simulink model "Polaris_demo"  (Simulink 9.2)
settings: Solver=FixedStepDiscrete  StartTime=0.0  StopTime=Inf  RelTol=1e-3  EnableMultiTasking=on
libraries: rpi_blkst x2
settings Model: Creator=jacques  LastModifiedBy=jacques  SimulationMode=external
settings OptimizationCC: ExpressionDepthLimit=2147483647  LifeSpan=1
settings DebuggingCC: SolverPrmCheckMsg=warning
settings HardwareCC: ProdLargestAtomicInteger=Long  ProdLargestAtomicFloat=Double  ProdIntDivRoundTo=Zero  ProdEndianess=LittleEndian  ProdHWDeviceType=ARM Compatible->ARM Cortex
settings SFSimCC: MATLABDynamicMemAlloc=off
settings RTWCC: SystemTargetFile=ert_rpi.tlc  TemplateMakefile=ert_rpi.tmf  PostCodeGenCommand=postGenFunc(buildInfo)  Description=RTW Embedded Coder RPI target
settings CodeAppCC: IgnoreCustomStorageClasses=off  CustomSymbolStrType=$N$R$M  InternalIdentifier=Classic
settings STFCustomTargetCC: ModelReferenceCompliant=off  CombineOutputUpdateFcns=on  ERTCustomFileBanners=on  SupportNonInlinedSFcns=off  RemoveResetFunc=on  MATLABClassNameForMDSCustomization=Simulink.SoftwareTarget.ERTCustomization  GRTInterface=off  SystemTargetFile=ert_rpi.tlc
settings ERTTargetCC: MultiwordLength=2048  ModelReferenceCompliant=off  ParMdlRefBuildCompliant=off  CompOptLevelCompliant=off  ConcurrentExecutionCompliant=off  SupportContinuousTime=on  ModelStepFunctionPrototypeControlCompliant=off  CPPClassGenCompliant=off  UseToolchainInfoCompliant=off  ExtMode=on  ExtModeMexArgs='192.168.2.1'  ERTCustomFileTemplate=ert_rpi_file_process.tlc  ConvertIfToSwitch=off  SuppressUnreachableDefaultCases=off

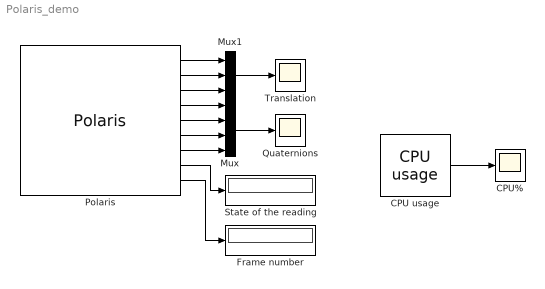
== system Polaris_demo ==
  CPU usage : rpi_blkst/CPU usage  rpi_mask_Ts=0.01
      settings: SourceProductName=RPI Blockset
  CPU% : Scope
  Frame number : Display
  Mux : Mux
  Mux1 : Mux  Inputs=3
  Polaris : rpi_blkst/Polaris  rpi_mask_Ts=0.01
      settings: SourceProductName=RPI Blockset
  Quaternions : Scope
  State of the reading : Display
  Translation : Scope
  wires:
  Polaris/9 -> Frame number/1
  Polaris/8 -> State of the reading/1
  Polaris/4 -> Mux/1
  Polaris/5 -> Mux/2
  Polaris/6 -> Mux/3
  Polaris/7 -> Mux/4
  Mux/1 -> Quaternions/1
  Polaris/2 -> Mux1/2
  Polaris/3 -> Mux1/3
  Polaris/1 -> Mux1/1
  Mux1/1 -> Translation/1
  CPU usage/1 -> CPU%/1
